simulink model "zygo_demo_status"  (Simulink 7.8)
settings: Solver=FixedStepDiscrete  StartTime=0.0  StopTime=inf  FixedStep=0.01  RelTol=1e-3
libraries: speedgoatlib_ZMI4104 x4, xpclib x3
settings Model: Creator=dkuratli  LastModifiedBy=lab3  BufferReuse=off
settings DataIOCC: SignalLoggingSaveFormat=Dataset
settings OptimizationCC: BlockReduction=off  OptimizeBlockIOStorage=off  BufferReuse=off  ExpressionFolding=off  LocalBlockOutputs=off
settings HardwareCC: ProdIntDivRoundTo=Zero  ProdEndianess=LittleEndian  ProdHWDeviceType=Generic->32-bit x86 compatible
settings RTWCC: SystemTargetFile=xpctarget.tlc  TemplateMakefile=xpc_default_tmf  Description=Simulink Real-Time  ProcessScript=xpctarget_make_rtw_hook  RTWCompilerOptimization=On
settings CodeAppCC: CustomSymbolStrType=$N$R$M_T
settings xpcTargetCC: TargetFcnLib=ansi_tfl_table_tmw.mat  TargetFunctionLibrary=XPC_BLAS  ParMdlRefBuildCompliant=on  ConcurrentExecutionCompliant=on  CombineSignalStateStructs=off  GRTInterface=on  GenerateAllocFcn=off  xPCTaskExecutionProfile=off  xPCRL32EventNumber=5000  xPCisModelTimeout=off  xPCModelTimeoutSecs=15  xPCLoadParamSetFile=off  xPCConcurrentTasks=off  xPCEnableSFAnimation=off

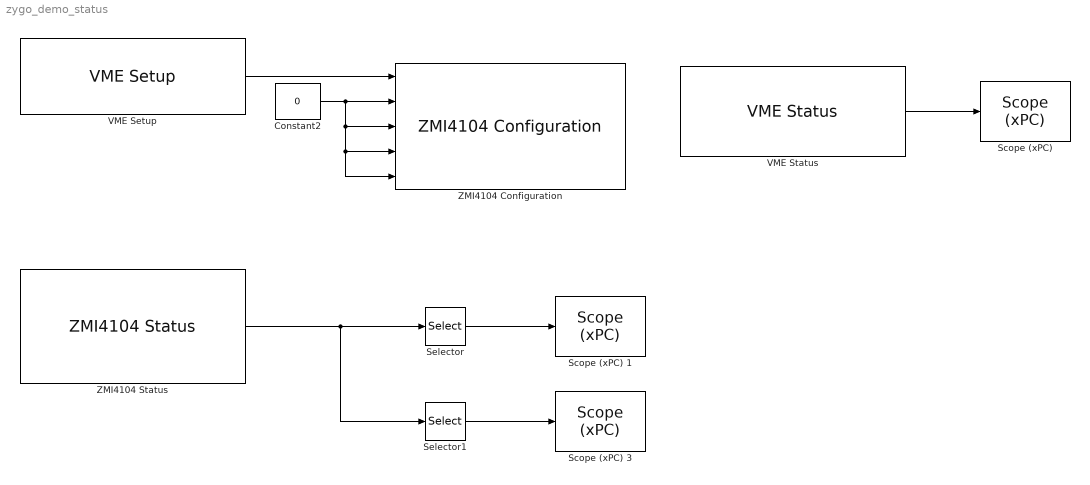
== system zygo_demo_status ==
  Constant2 : Constant  Value=0
  "Scope (xPC) " : xpclib/Misc./Scope (xPC)   scopeno=1  scopetype=Target  autostart=on  viewmode=Numerical  formatstr='VME link error: %1.0f'  grid=on  ylimits=[0,0]  nosamples=3  noprepostsamples=0  interleave=1  triggermode=FreeRun  triggersignal=1  trigsignalfromport=off  triggerlevel=0.0  triggerslope=Either  triggerscope=1  triggersample=0  filename=data.dat  mode=Lazy  writesize=512  autorestart=off  dynamicfilemode=off  maxwritefilesize=512*1024^2
  Scope (xPC) 1 : xpclib/Misc./Scope (xPC)   scopeno=2  scopetype=Target  autostart=on  viewmode=Numerical  formatstr='Power Error: %1.0f,Write Error: %1.0f,Reference Signal Missing: %1.0f,Reference PLL Error: %1.0f,Reset Complete: %1.0f,Reset Failure: %1.0f,FPGA Sync Error: %1.0f,OverTempError: %1.0f,Measure Signal Missing: %1.0f,Measure Signal Saturated: %1.0f'  grid=on  ylimits=[0,0]  nosamples=3  noprepostsamples=0  interleave=1  triggermode=FreeRun  triggersignal=1  trigsignalfromport=off  triggerlevel=0.0  triggerslope=Either  triggerscope=1  triggersample=0  filename=data.dat  mode=Lazy  writesize=512  autorestart=off  dynamicfilemode=off  maxwritefilesize=512*1024^2
  Scope (xPC) 3 : xpclib/Misc./Scope (xPC)   scopeno=3  scopetype=Target  autostart=on  viewmode=Numerical  formatstr='SSI Max Limit: %1.0f,Measure Signal Dropout: %1.0f,Measure Signal Glitch: %1.0f,Acceleration Error: %1.0f,Phase Noise Error: %1.0f,CEC Error: %1.0f,Velocity Error: %1.0f,User Velocity Error: %1.0f,37-bit Position Overflow: %1.0f,VME 32 bit Position Overflow: %1.0f'  grid=on  ylimits=[0,0]  nosamples=3  noprepostsamples=0  interleave=1  triggermode=FreeRun  triggersignal=1  trigsignalfromport=off  triggerlevel=0.0  triggerslope=Either  triggerscope=1  triggersample=0  filename=data.dat  mode=Lazy  writesize=512  autorestart=off  dynamicfilemode=off  maxwritefilesize=512*1024^2
  Selector : Selector  InputPortWidth=20  Indices=[1,2,3,4,5,6,7,8,9,10]
  Selector1 : Selector  InputPortWidth=20  Indices=[11,12,13,14,15,16,17,18,19,20]
  VME Setup : speedgoatlib_ZMI4104/VME Setup  id=1  modules=1  slot=-1  z1_id=1  z1_addr_sw1=0  z1_addr_sw2=0  z2_id=2  z2_addr_sw1=0  z2_addr_sw2=1
  VME Status : speedgoatlib_ZMI4104/VME Status  id=1  ts=-1  slot=-1
  ZMI4104 Configuration : speedgoatlib_ZMI4104/ZMI4104 Configuration  id=1  ts=-1  slot=-1  ax1_filter_kv=-19  ax1_filter_kp=-8  ax2_filter_kv=-19  ax2_filter_kp=-8  ax3_filter_kv=-19  ax3_filter_kp=-8  ax4_filter_kv=-19  ax4_filter_kp=-8
  ZMI4104 Status : speedgoatlib_ZMI4104/ZMI4104 Status  id=1  zmi_id=1  axis=1  ts=-1  slot=-1
  wires:
  VME Setup/1 -> ZMI4104 Configuration/1
  Constant2/1 -> ZMI4104 Configuration/2, ZMI4104 Configuration/5, ZMI4104 Configuration/4, ZMI4104 Configuration/3
  VME Status/1 -> "Scope (xPC) "/1
  Selector/1 -> Scope (xPC) 1/1
  Selector1/1 -> Scope (xPC) 3/1
  ZMI4104 Status/1 -> Selector/1, Selector1/1
